simulink model "SistemaIdraulico"  (R2013b)
settings: Solver=ode23tb  StartTime=0.0  StopTime=3  MaxStep=0.00001  RelTol=1e-3
values from neighbouring files (symbols this model uses):
  A1 = get(handles.A1, 'Value')    [Main.m]
  A2 = get(handles.A2, 'Value')    [Main.m]
  h10 = get(handles.h10, 'Value')    [Main.m]
  h20 = get(handles.h20, 'Value')    [Main.m]
  Mur1 = get(handles.Mur1, 'Value')    [Main.m]
  R1 = get(handles.R1, 'Value')    [Main.m]
  R2 = get(handles.R2, 'Value')    [Main.m]
  rho = get(handles.rho, 'Value')    [Main.m]
  Sph1 = get(handles.Sph1, 'Value')    [Main.m]
settings Model: Creator=alex  LastModifiedBy=Giorgia Adorni
settings OptimizationCC: ExpressionDepthLimit=2147483647  InitFltsAndDblsToZero=on
settings DebuggingCC: SaveWithParameterizedLinksMsg=none  SolverPrmCheckMsg=none  FcnCallInpInsideContextMsg=UseLocalSettings  StateNameClashWarn=warning
settings GRTTargetCC: TargetFcnLib=ansi_tfl_tmw.mat  CombineOutputUpdateFcns=off  GRTInterface=on

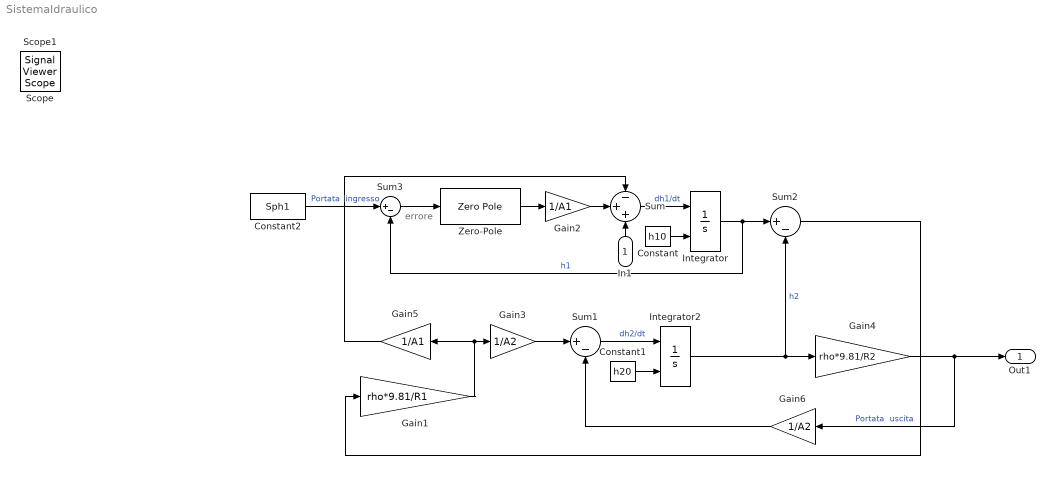
== system SistemaIdraulico ==
  note: errore
  In1 : Inport
  Constant : Constant  Value=h10
  Constant1 : Constant  Value=h20
  Constant2 : Constant  Value=Sph1
  Gain1 : Gain  Gain=rho*9.81/R1
  Gain2 : Gain  Gain=1/A1
  Gain3 : Gain  Gain=1/A2
  Gain4 : Gain  Gain=rho*9.81/R2
  Gain5 : Gain  Gain=1/A1
  Gain6 : Gain  Gain=1/A2
  Integrator : Integrator  InitialConditionSource=external
  Integrator2 : Integrator  InitialConditionSource=external
  Sum : Sum  Inputs=-++
  Sum1 : Sum  Inputs=|+-
  Sum2 : Sum  Inputs=|+-
  Sum3 : Sum  Inputs=|+-
  Zero-Pole : ZeroPole  Zeros=[-2 -10]  Poles=[-8 -0.1]  Gain=Mur1
  Out1 : Outport
  Scope : SignalViewerScope  IOType=viewer  RefreshTime=0.035000
      settings: YMin=0
  Scope1 : SignalViewerScope  IOType=viewer  NumInputPorts=4  ZoomMode=xonly  RefreshTime=0.037936
      settings: YMin=4.75~0~0~0  YMax=5.25~5.5~2.75~55
  wires:
  Sum/1 -> Integrator/1  "dh1/dt"
  Gain1/1 -> Gain5/1, Gain3/1
  Gain4/1 -> Out1/1, Gain6/1  "Portata  uscita"
  Integrator2/1 -> Gain4/1, Sum2/2  "h2"
  Sum1/1 -> Integrator2/1  "dh2/dt"
  In1/1 -> Sum/3
  Constant/1 -> Integrator/2
  Constant1/1 -> Integrator2/2
  Constant2/1 -> Sum3/1  "Portata  ingresso"
  Gain2/1 -> Sum/2
  Integrator/1 -> Sum2/1, Sum3/2  "h1"
  Gain5/1 -> Sum/1
  Gain6/1 -> Sum1/2
  Sum2/1 -> Gain1/1
  Zero-Pole/1 -> Gain2/1
  Sum3/1 -> Zero-Pole/1
  Gain3/1 -> Sum1/1
